simulink model "QuarterCar_2DOF"  (R2025b)
settings: Solver=VariableStepAuto  StartTime=0.0  StopTime=10.0  RelTol=1e-3
settings Model: Creator=Aditya  LastModifiedBy=Aditya

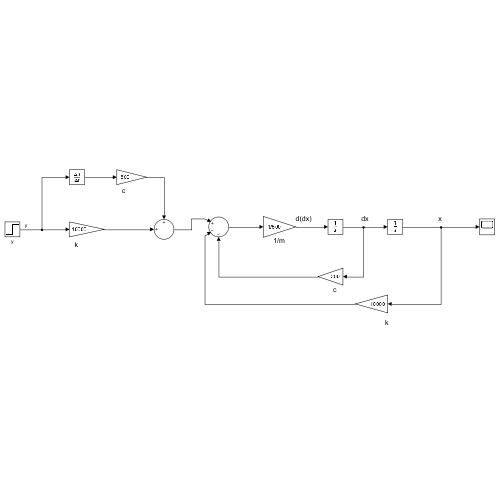
[thumbnail: Simulink's stored preview of the top-level diagram]
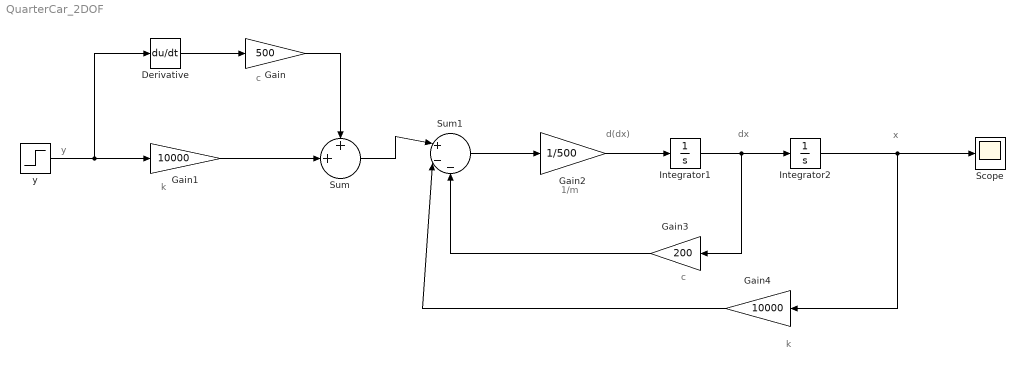
== system QuarterCar_2DOF ==
  note: y
  note: k
  note: d(dx)
  note: dx
  note: x
  note: c
  note: k
  note: c
  note: 1/m
  Derivative : Derivative
  Gain : Gain  Gain=500
  Gain1 : Gain  Gain=10000
  Gain2 : Gain  Gain=1/500
  Gain3 : Gain  Gain=200
  Gain4 : Gain  Gain=10000
  Integrator1 : Integrator
  Integrator2 : Integrator
  Scope : Scope
  Sum : Sum  Inputs=++|
  Sum1 : Sum  Inputs=|+--
  y : Step  Time=0.1  SampleTime=0
  wires:
  y/1 -> Derivative/1, Gain1/1
  Derivative/1 -> Gain/1
  Sum/1 -> Sum1/1
  Sum1/1 -> Gain2/1
  Gain2/1 -> Integrator1/1
  Integrator1/1 -> Gain3/1, Integrator2/1
  Integrator2/1 -> Gain4/1, Scope/1
  Gain3/1 -> Sum1/3
  Gain4/1 -> Sum1/2
  Gain/1 -> Sum/1
  Gain1/1 -> Sum/2
